simulink model "B_robustness_Tracking_Integral_for_second_desired_poles"  (R2021b)
settings: Solver=VariableStepAuto  StartTime=0.0  StopTime=0.5  RelTol=1e-3
undefined symbols (not defined in the file): A, B_r, KI2_1, KI2_2
settings Model: Creator=nima8  LastModifiedBy=nima8

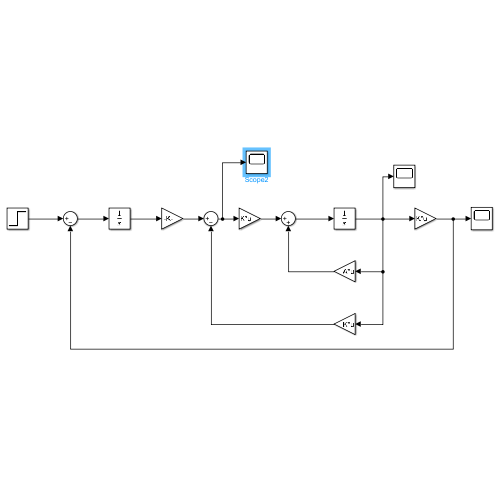
[thumbnail: Simulink's stored preview of the top-level diagram]
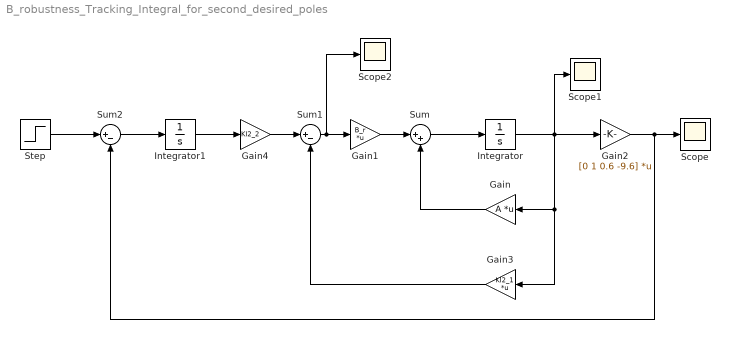
== system B_robustness_Tracking_Integral_for_second_desired_poles ==
  Gain : Gain  Gain=A  Multiplication=Matrix(K*u)
  Gain1 : Gain  Gain=B_r  Multiplication=Matrix(K*u)
  Gain2 : Gain  Gain=[0 1 0.6 -9.6]  Multiplication=Matrix(K*u)
  Gain3 : Gain  Gain=KI2_1  Multiplication=Matrix(K*u)
  Gain4 : Gain  Gain=KI2_2
  Integrator : Integrator  InitialCondition=[1 0.5 -1 2]
  Integrator1 : Integrator  InitialCondition=2
  Scope : Scope
  Scope1 : Scope
  Scope2 : Scope
  Step : Step  Time=0  SampleTime=0
  Sum : Sum  Inputs=|++
  Sum1 : Sum  Inputs=|+-
  Sum2 : Sum  Inputs=|+-
  wires:
  Step/1 -> Sum2/1
  Integrator/1 -> Scope1/1, Gain/1, Gain3/1, Gain2/1
  Gain2/1 -> Sum2/2, Scope/1
  Sum1/1 -> Scope2/1, Gain1/1
  Gain3/1 -> Sum1/2
  Gain/1 -> Sum/2
  Gain1/1 -> Sum/1
  Integrator1/1 -> Gain4/1
  Sum/1 -> Integrator/1
  Sum2/1 -> Integrator1/1
  Gain4/1 -> Sum1/1
